simulink model "sim_relay_system"  (R2019a)
settings: Solver=FixedStepAuto  StartTime=0.0  StopTime=end_time  FixedStep=FStep  RelTol=1e-3  EnableMultiTasking=on
undefined symbols (not defined in the file): d, h, K, T, x0, y0, z0
libraries: simulink_extras x1
settings Model: Creator=user  LastModifiedBy=ogure
settings SolverCC: SolverResetMethod=Robust
settings DataIOCC: LimitDataPoints=on  SaveFormat=Array  SaveOutput=off  ReturnWorkspaceOutputs=off  OutputSaveName=X,X1,X2,X3,X4,L,H
settings OptimizationCC: LifeSpan=inf
settings DebuggingCC: SolverPrmCheckMsg=warning  SFUnexpectedBacktrackingDiag=warning  SFNoUnconditionalDefaultTransitionDiag=warning  SFExecutionAtInitializationDiag=none  ArithmeticOperatorsInVariantConditions=warning
settings HardwareCC: ProdBitPerPointer=32  ProdBitPerSizeT=32  ProdBitPerPtrDiffT=32  ProdLargestAtomicFloat=None  ProdIntDivRoundTo=Undefined  ProdEndianess=Unspecified  ProdWordSize=32  ProdHWDeviceType=32-bit Generic
settings ModelReferenceCC: PropagateSignalLabelsOutOfModel=off
settings SFSimCC: SimUseLocalCustomCode=off
settings RTWCC: RTWUseLocalCustomCode=off
settings CodeAppCC: StateflowObjectComments=on
settings GRTTargetCC: TargetLangStandard=C89/C90 (ANSI)  GeneratePreprocessorConditionals=Disable all
settings ConfigComp: CovMetricSettings=dw  CovHtmlReporting=on  CovSaveCumulativeToWorkspaceVar=on  CovSaveSingleToWorkspaceVar=on  CovExternalEMLEnable=off  CovSFcnEnable=off

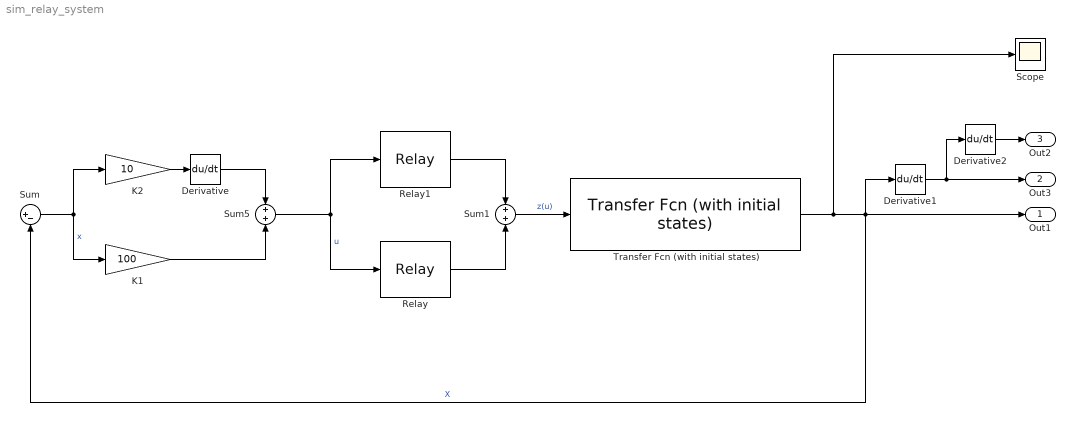
== system sim_relay_system ==
  Derivative : Derivative  CoefficientInTFapproximation=0.00000001
  Derivative1 : Derivative  CoefficientInTFapproximation=0.00000001
  Derivative2 : Derivative  CoefficientInTFapproximation=0.00000001
  K1 : Gain  Gain=100
  "K2 " : Gain  Gain=10
  Relay : Relay  OnSwitchValue=d  OffSwitchValue=d  OnOutputValue=d
  Relay1 : Relay  OnSwitchValue=-d  OffSwitchValue=-d  OnOutputValue=0  OffOutputValue=-d
  Scope : Scope
  Sum : Sum  Inputs=|+-
  Sum1 : Sum
  Sum5 : Sum
  Transfer Fcn (with initial states) : simulink_extras/Additional Linear/Transfer Fcn (with initial states)  N=K  D=[T^2 2*h*T 1 0]  X0=[z0 y0 x0]
  Out1 : Outport  SignalName=X
  Out3 : Outport  Port=2  SignalName=y
  Out2 : Outport  Port=3  SignalName=z
  wires:
  Transfer Fcn (with initial states)/1 -> Scope/1, Sum/2, Derivative1/1, Out1/1  "X"
  Sum5/1 -> Relay1/1, Relay/1  "u"
  Sum1/1 -> Transfer Fcn (with initial states)/1  "z(u)"
  Derivative/1 -> Sum5/1
  K1/1 -> Sum5/2
  Sum/1 -> K1/1, "K2 "/1  "x"
  "K2 "/1 -> Derivative/1
  Relay1/1 -> Sum1/1
  Relay/1 -> Sum1/2
  Derivative1/1 -> Derivative2/1, Out3/1
  Derivative2/1 -> Out2/1
